simulink model "VTOL_sim"  (R2016b)
settings: Solver=ode45  StartTime=0.0  StopTime=10000  RelTol=1e-3  EnableMultiTasking=on
InitFcn:
  | addpath ./..
  | VTOL_param
undefined symbols (not defined in the file): P, VTOL_animation
libraries: simulink x1
settings Model: Creator=beard  LastModifiedBy=beard
settings DataIOCC: LimitDataPoints=on  SaveFormat=Array  SignalLoggingSaveFormat=ModelDataLogs
settings OptimizationCC: ExpressionDepthLimit=2147483647  InitFltsAndDblsToZero=on  LifeSpan=inf
settings DebuggingCC: UnderspecifiedInitializationDetection=Classic  MergeDetectMultiDrivingBlocksExec=none  SolverPrmCheckMsg=warning  FcnCallInpInsideContextMsg=warning  StateNameClashWarn=warning  SFUnexpectedBacktrackingDiag=warning  SFNoUnconditionalDefaultTransitionDiag=warning  SFExecutionAtInitializationDiag=none
settings HardwareCC: ProdBitPerPointer=32  ProdBitPerSizeT=32  ProdBitPerPtrDiffT=32  ProdLargestAtomicFloat=None  ProdIntDivRoundTo=Undefined  ProdEndianess=Unspecified  ProdWordSize=32  ProdHWDeviceType=32-bit Generic
settings ModelReferenceCC: PropagateSignalLabelsOutOfModel=off
settings GRTTargetCC: TargetLangStandard=C89/C90 (ANSI)  GeneratePreprocessorConditionals=Disable all  CombineOutputUpdateFcns=off  GRTInterface=on
settings ConfigComp: CovMetricSettings=dw  CovHtmlReporting=on  CovSaveCumulativeToWorkspaceVar=on  CovSaveSingleToWorkspaceVar=on  CovExternalEMLEnable=off

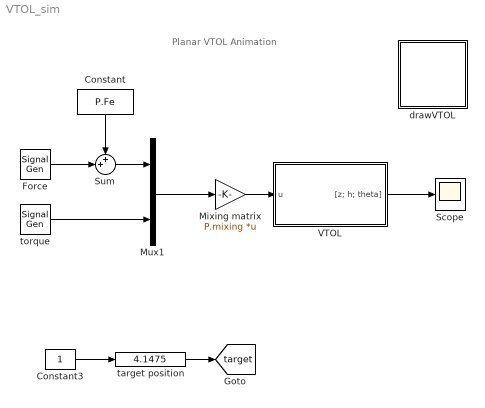
== system VTOL_sim ==
  note: Planar VTOL Animation
  Constant : Constant  Value=P.Fe
  Constant3 : Constant
  Force : SignalGenerator  Amplitude=.1  Frequency=.1
  Mixing matrix : Gain  Gain=P.mixing  Multiplication=Matrix(K*u)
  Mux1 : Mux  Inputs=2
  Scope : Scope
  Sum : Sum  Inputs=++|
  VTOL : Subsystem
  drawVTOL : Subsystem
      mask Display: image(imread('tv.jpg'))
  target position : simulink/Math Operations/Slider Gain  low=0  gain=4.1475  high=6
  torque : SignalGenerator  Amplitude=.01  Frequency=2
  tag scope: target=global
  wires:
  Constant3/1 -> target position/1
  target position/1 -> [target]
  VTOL/1("[z; h; theta]") -> Scope/1
  Constant/1 -> Sum/1
  Sum/1 -> Mux1/1
  torque/1 -> Mux1/2
  Force/1 -> Sum/2
  Mixing matrix/1 -> VTOL/1(u)
  Mux1/1 -> Mixing matrix/1

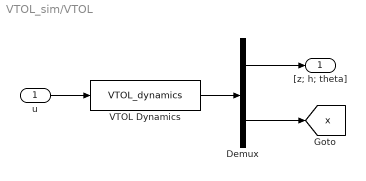
== system VTOL_sim/VTOL ==
  u : Inport
  Demux : Demux  Outputs=[3;6]
  VTOL Dynamics : S-Function  FunctionName=VTOL_dynamics  Parameters=P  SFunctionDeploymentMode=off  EnableBusSupport=off
  "[z; h; theta]" : Outport
  tag scope: x=global
  wires:
  u/1 -> VTOL Dynamics/1
  VTOL Dynamics/1 -> Demux/1
  Demux/1 -> "[z; h; theta]"/1
  Demux/2 -> [x]

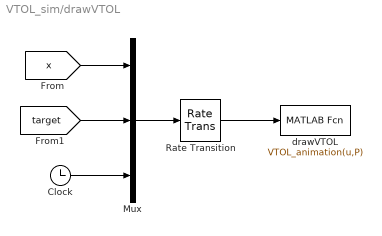
== system VTOL_sim/drawVTOL ==
  Clock : Clock
  Mux : Mux  Inputs=3
  Rate Transition : RateTransition  OutPortSampleTime=P.t_plot
  drawVTOL : MATLABFcn  MATLABFcn=VTOL_animation(u,P)  OutputDimensions=0
  wires:
  Mux/1 -> Rate Transition/1
  [x] -> Mux/1
  Clock/1 -> Mux/3
  Rate Transition/1 -> drawVTOL/1
  [target] -> Mux/2
